simulink model "RSC_RRT"  (R2012b)
settings: Solver=ode3  StartTime=0.0  StopTime=10  FixedStep=.05  RelTol=1e-3
InitFcn:
  | a2g = 1/9.81;
  | r2d = 180/pi;
  | K_sr = 15.97;
  | neutral_steer = 104;
  | s2t = (pi/180)*(1/K_sr);
  | A_kt =[         0         0         0         0         0         0
  |          0   -3.5058   -1.6990  -25.6114   -2.2435         0
  |          0    2.2782   -4.2575  -64.1772   -5.6218         0
  |          0         0    1.0000         0         0         0
  |          0   -0.0158    0.0295    0.4442   -4.1900         0
  |          0         0         0         0    1.0000         0];
  | 
  | 
  | B_kt =[0
  |    23.7845
  |   -16.0342
  |          0
  |    17.5770
  |          0];
  | 
  | load MPC_test_2
undefined symbols (not defined in the file or in its folder): CR, DiscIntNeverNeededParam, serial
libraries: instrumentlib x3, mpclib x1, simulink x1, realtime_pacer_lib x1
settings Model: BufferReuse=off  Creator=TCA  LastModifiedBy=Thomas
settings DataIOCC: SignalLoggingSaveFormat=ModelDataLogs
settings OptimizationCC: BlockReduction=off  InlineParams=on  BufferReuse=off  InitFltsAndDblsToZero=on
settings DebuggingCC: ReadBeforeWriteMsg=DisableAll  AlgebraicLoopMsg=none  SolverPrmCheckMsg=none  FcnCallInpInsideContextMsg=UseLocalSettings  UnconnectedInputMsg=none  UnconnectedOutputMsg=none  UnconnectedLineMsg=none  StrictBusMsg=Warning
settings SFSimCC: SimParseCustomCode=off
settings RTWCC: TargetLang=C++
settings GRTTargetCC: CombineOutputUpdateFcns=off  GRTInterface=on

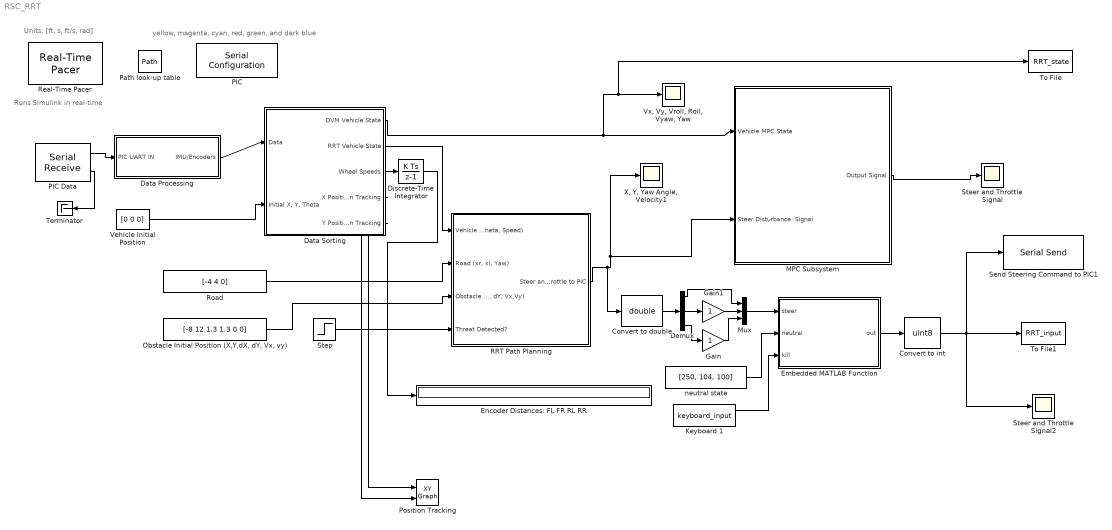
== system RSC_RRT ==
  note: Runs Simulink
      |  in real-time
  note: Units: [ft, s, ft/s, rad]
  note: yellow, magenta, cyan, red, green, and dark blue
  Convert to double : DataTypeConversion  OutDataTypeStr=double  SampleTime=0.05  SaturateOnIntegerOverflow=on  RndMeth=Zero
  Convert to int : DataTypeConversion  OutDataTypeStr=uint8  SampleTime=0.05  SaturateOnIntegerOverflow=on  RndMeth=Zero
  Data Processing : Subsystem
  Data Sorting : Subsystem
  Demux : Demux  Outputs=3
  Discrete-Time Integrator : DiscreteIntegrator  SampleTime=0.05  ICPrevOutput=DiscIntNeverNeededParam  ICPrevScaledInput=DiscIntNeverNeededParam
  Embedded MATLAB Function : MATLAB Function  TreatAsAtomicUnit=on
  Encoder Distances: FL FR RL RR : Display
  Gain : Gain
  Gain1 : Gain
  Keyboard 1 : M-S-Function  FunctionName=keyboard_input  mask(Keyboard Input){}
      mask help: Keyboard Input
      mask Display: fprintf('Keyboard');
  MPC Subsystem : Subsystem
  Mux : Mux  Inputs=3
  "Obstacle Initial Position (X,Y,dX, dY, Vx, vy)" : Constant  Value=[-8 12 1.3 1.3 0 0]
  PIC : instrumentlib/Serial Configuration  Priority=-200000  ComPortMenu=<Please select a port...>  ComPort=COM5  ObjConstructor=serial('COM5');  BaudRate=9600  DataBits=8  Parity=none  StopBits=1  FlowControl=none  Timeout=10  ByteOrder=LittleEndian
  PIC Data : instrumentlib/Serial Receive  ComPortMenu=<Please select a port...>  ComPort=COM5  ObjConstructor=serial('COM5');  Terminator=CR ('\r')  DataSize="[1  16]"  DataType=uint8  EnableBlockingMode=off  ActionDataUnavailable=Output last received value  CustomValue=0  SampleTime=.05
  Path look-up table : DataStoreMemory  DataStoreName=Path  ReadBeforeWriteMsg=warning  WriteAfterWriteMsg=warning  WriteAfterReadMsg=warning  InitialValue=zeros(50, 6)  VectorParams1D=off
  Position Tracking : simulink/Sinks/XY Graph  xmin=-10  xmax=10  ymin=-10  ymax=50  st=-1
  RRT Path Planning : Subsystem
  Real-Time Pacer : realtime_pacer_lib/Real-Time Pacer  simTimePerRealTime=1
  Road : Constant  Value=[-4 4 0]
  Send Steering Command to PIC1 : instrumentlib/Serial Send  ComPortMenu=<Please select a port...>  ComPort=COM5  ObjConstructor=serial('COM5');  Header=250  Terminator=<none>  EnableBlockingMode=off
  Steer and Throttle Signal : Scope
      settings: TimeRange=10  YMin=50  YMax=250  SaveName=ScopeData3
  Steer and Throttle Signal2 : Scope
      settings: TimeRange=10  YMin=50  YMax=250  SaveName=ScopeData4
  Step : Step  Time=2  SampleTime=0
  Terminator : Terminator
  To File : ToFile  Filename=RRT_state  MatrixName=RRT_state  SaveFormat=Timeseries
  To File1 : ToFile  Filename=RRT_input  MatrixName=RRT_input  SaveFormat=Timeseries
  Vehicle Initial Position : Constant  Value=[0 0 0]  VectorParams1D=off
  "Vx, Vy, Vroll, Roll, Vyaw, Yaw" : Scope
      settings: TimeRange=10  YMax=30  SaveName=ScopeData2
  "X, Y, Yaw Angle, Velocity1" : Scope
      settings: TimeRange=10  YMax=30  SaveName=ScopeData6
  neutral state : Constant  Value=[250, 104, 100]
  wires:
  PIC Data/2 -> Terminator/1
  Vehicle Initial Position/1 -> Data Sorting/2("Initial X, Y, Theta")
  PIC Data/1 -> Data Processing/1(PIC UART IN)
  Data Processing/1(IMU/Encoders) -> Data Sorting/1(Data)
  Discrete-Time Integrator/1 -> Encoder Distances: FL FR RL RR/1
  Data Sorting/3(Wheel Speeds) -> Discrete-Time Integrator/1
  Data Sorting/4(X Position Tracking) -> Position Tracking/1
  Data Sorting/5(Y Position Tracking) -> Position Tracking/2
  Data Sorting/1(DVM Vehicle State) -> MPC Subsystem/1(Vehicle MPC State), "Vx, Vy, Vroll, Roll, Vyaw, Yaw"/1, To File/1
  MPC Subsystem/1(Output Signal) -> Steer and Throttle Signal/1
  RRT Path Planning/1(Steer and Throttle to PIC) -> "X, Y, Yaw Angle, Velocity1"/1, MPC Subsystem/2(Steer Disturbance  Signal), Convert to double/1
  neutral state/1 -> Embedded MATLAB Function/2(neutral)
  Keyboard 1/1 -> Embedded MATLAB Function/3(kill)
  Embedded MATLAB Function/1(out) -> Convert to int/1
  Convert to int/1 -> Send Steering Command to PIC1/1, To File1/1, Steer and Throttle Signal2/1
  Convert to double/1 -> Demux/1
  Demux/3 -> Gain/1
  Gain/1 -> Mux/3
  Demux/1 -> Mux/1
  Mux/1 -> Embedded MATLAB Function/1(steer)
  Demux/2 -> Gain1/1
  Gain1/1 -> Mux/2
  Step/1 -> RRT Path Planning/4(Threat Detected?)
  "Obstacle Initial Position (X,Y,dX, dY, Vx, vy)"/1 -> RRT Path Planning/3("Obstacle Array (X,Y,dX, dY, Vx,Vy)")
  Road/1 -> RRT Path Planning/2("Road (xr, xl, Yaw)")
  Data Sorting/2(RRT Vehicle State) -> RRT Path Planning/1("Vehicle State (X,Y, Theta, Speed)")

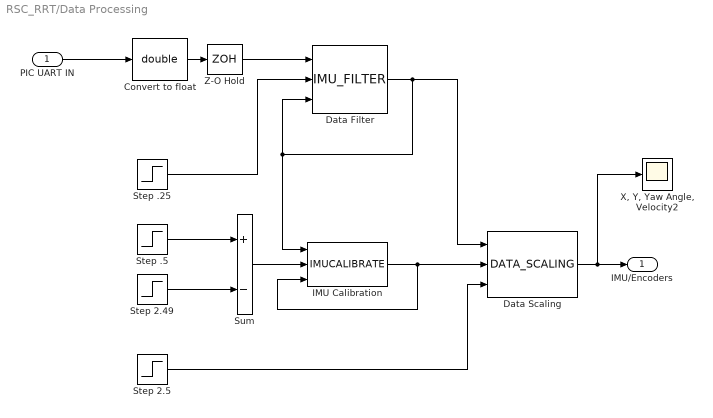
== system RSC_RRT/Data Processing ==
  PIC UART IN : Inport
  Convert to float : DataTypeConversion  OutDataTypeStr=double  SaturateOnIntegerOverflow=on  RndMeth=Zero
  Data Filter : M-S-Function  FunctionName=IMU_FILTER  Parameters=3
  "Data Scaling " : M-S-Function  FunctionName=DATA_SCALING  Parameters=3
  IMU Calibration : M-S-Function  FunctionName=IMUCALIBRATE  Parameters=3
  Step .25 : Step  Time=.25  SampleTime=0
  Step .5 : Step  Time=.5  SampleTime=0
  Step 2.49 : Step  Time=2.49  SampleTime=0
  Step 2.5 : Step  Time=2.5  SampleTime=0
  Sum : Sum  Inputs=+-
  "X, Y, Yaw Angle, Velocity2" : Scope
      settings: TimeRange=10  YMax=30  SaveName=ScopeData9
  Z-O Hold : ZeroOrderHold  SampleTime=0.05
  IMU/Encoders : Outport
  wires:
  Convert to float/1 -> Z-O Hold/1
  Data Filter/1 -> "Data Scaling "/1, IMU Calibration/1, Data Filter/3
  IMU Calibration/1 -> IMU Calibration/3, "Data Scaling "/2
  Step .5/1 -> Sum/1
  Step 2.49/1 -> Sum/2
  Z-O Hold/1 -> Data Filter/1
  Step .25/1 -> Data Filter/2
  Sum/1 -> IMU Calibration/2
  Step 2.5/1 -> "Data Scaling "/3
  "Data Scaling "/1 -> IMU/Encoders/1, "X, Y, Yaw Angle, Velocity2"/1
  PIC UART IN/1 -> Convert to float/1

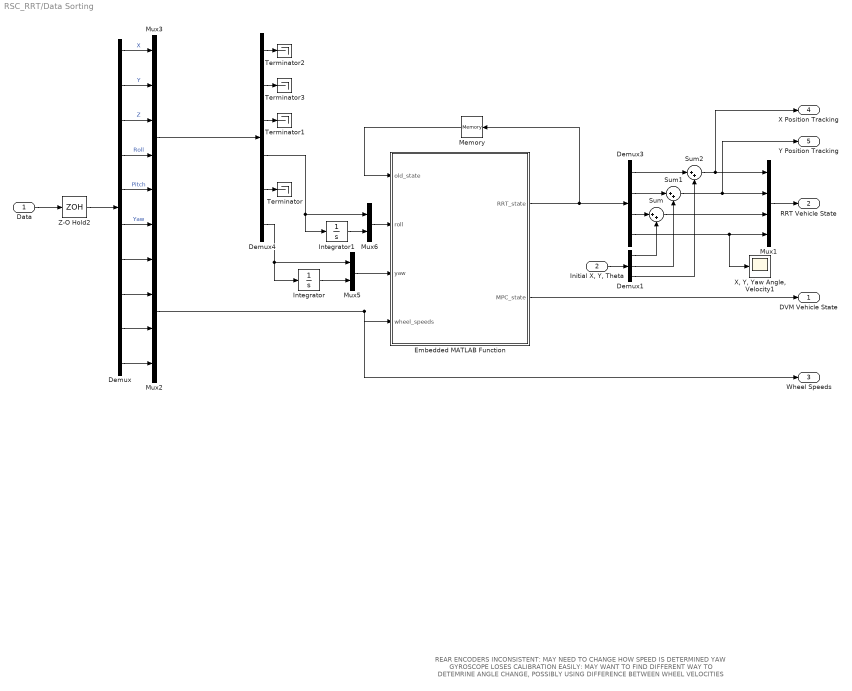
== system RSC_RRT/Data Sorting ==
  note: REAR ENCODERS INCONSISTENT: MAY NEED TO CHANGE HOW SPEED IS DETERMINED
      | YAW GYROSCOPE LOSES CALIBRATION EASILY: MAY WANT TO FIND DIFFERENT WAY TO DETEMRINE
      | ANGLE CHANGE, POSSIBLY USING DIFFERENCE BETWEEN WHEEL VELOCITIES
  Data : Inport
  "Initial X, Y, Theta" : Inport  Port=2
  Demux : Demux  Outputs=10
  Demux1 : Demux  Outputs=3
  Demux3 : Demux
  Demux4 : Demux  Outputs=6
  Embedded MATLAB Function : MATLAB Function  TreatAsAtomicUnit=on
  Integrator : Integrator
  Integrator1 : Integrator
  Memory : Memory  InheritSampleTime=on
  Mux1 : Mux
  Mux2 : Mux
  Mux3 : Mux  Inputs=6
  Mux5 : Mux  Inputs=2
  Mux6 : Mux  Inputs=2
  Sum : Sum  Inputs=|++
  Sum1 : Sum  Inputs=|++
  Sum2 : Sum  Inputs=|++
  Terminator{,1..3} (4 alike) : Terminator
  "X, Y, Yaw Angle, Velocity1" : Scope
      settings: TimeRange=10  YMax=30  SaveName=ScopeData7
  Z-O Hold2 : ZeroOrderHold  SampleTime=0.05
  DVM Vehicle State : Outport
  RRT Vehicle State : Outport  Port=2
  Wheel Speeds : Outport  Port=3
  X Position Tracking : Outport  Port=4
  Y Position Tracking : Outport  Port=5
  wires:
  Data/1 -> Z-O Hold2/1
  "Initial X, Y, Theta"/1 -> Demux1/1
  Memory/1 -> Embedded MATLAB Function/1(old_state)
  Embedded MATLAB Function/1(RRT_state) -> Memory/1, Demux3/1
  Demux/6 -> Mux3/6  "Yaw"
  Demux/1 -> Mux3/1  "X"
  Demux/2 -> Mux3/2  "Y"
  Mux3/1 -> Demux4/1
  Demux/3 -> Mux3/3  "Z"
  Demux/4 -> Mux3/4  "Roll"
  Demux/5 -> Mux3/5  "Pitch"
  Demux/7 -> Mux2/1
  Demux/8 -> Mux2/2
  Demux/9 -> Mux2/3
  Demux/10 -> Mux2/4
  Mux2/1 -> Embedded MATLAB Function/4(wheel_speeds), Wheel Speeds/1
  Z-O Hold2/1 -> Demux/1
  Demux1/1 -> Sum/2
  Demux1/2 -> Sum1/2
  Demux1/3 -> Sum2/2
  Demux3/2 -> Sum1/1
  Demux3/1 -> Sum2/1
  Demux3/3 -> Sum/1
  Sum2/1 -> Mux1/1, X Position Tracking/1
  Sum1/1 -> Mux1/2, Y Position Tracking/1
  Sum/1 -> Mux1/3
  Mux1/1 -> RRT Vehicle State/1
  Demux3/4 -> Mux1/4, "X, Y, Yaw Angle, Velocity1"/1
  Demux4/4 -> Integrator1/1, Mux6/1
  Demux4/6 -> Integrator/1, Mux5/1
  Integrator/1 -> Mux5/2
  Mux5/1 -> Embedded MATLAB Function/3(yaw)
  Integrator1/1 -> Mux6/2
  Mux6/1 -> Embedded MATLAB Function/2(roll)
  Demux4/5 -> Terminator/1
  Demux4/3 -> Terminator1/1
  Demux4/1 -> Terminator2/1
  Demux4/2 -> Terminator3/1
  Embedded MATLAB Function/2(MPC_state) -> DVM Vehicle State/1

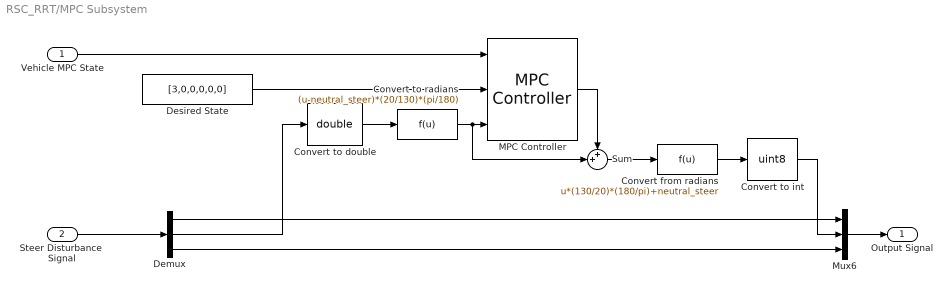
== system RSC_RRT/MPC Subsystem ==
  Vehicle MPC State : Inport
  Steer Disturbance  Signal : Inport  Port=2
  Convert from radians : Fcn  Expr=u*(130/20)*(180/pi)+neutral_steer
  Convert to double : DataTypeConversion  OutDataTypeStr=double  SampleTime=0.05  SaturateOnIntegerOverflow=on  RndMeth=Zero
  Convert to int : DataTypeConversion  OutDataTypeStr=uint8  SampleTime=0.05  SaturateOnIntegerOverflow=on  RndMeth=Zero
  Convert to radians : Fcn  Expr=(u-neutral_steer)*(20/130)*(pi/180)
  Demux : Demux  Outputs=3
  Desired State : Constant  Value=[3,0,0,0,0,0]
  MPC Controller : mpclib/MPC Controller  mpcobj=MPC_test_2  x0=[]  md_inport=on  mv_inport=off  lims_inport=off  switch_inport=off  ywt_inport=off  duwt_inport=off  rhoeps_inport=off  cost_outport=off  return_sequence=off  return_qpstatus=off  is_multiple=0  enable_value=0  n_mv=1  n_mo=6  n_md=1  n_ts=0.05  is_designfromscratch=0  ref_from_ws=off  ref_signal_name=[]  ref_preview=on  md_from_ws=off  md_signal_name=[]  md_preview=on  from_project=off  project_file=MPCtask.mat
  Mux6 : Mux  Inputs=3
  Sum : Sum  Inputs=++|
  Output Signal : Outport
  wires:
  Convert to double/1 -> Convert to radians/1
  Desired State/1 -> MPC Controller/2
  Convert to radians/1 -> MPC Controller/3, Sum/2
  MPC Controller/1 -> Sum/1
  Steer Disturbance  Signal/1 -> Demux/1
  Demux/2 -> Convert to double/1
  Demux/1 -> Mux6/1
  Convert from radians/1 -> Convert to int/1
  Demux/3 -> Mux6/3
  Mux6/1 -> Output Signal/1
  Vehicle MPC State/1 -> MPC Controller/1
  Sum/1 -> Convert from radians/1
  Convert to int/1 -> Mux6/2

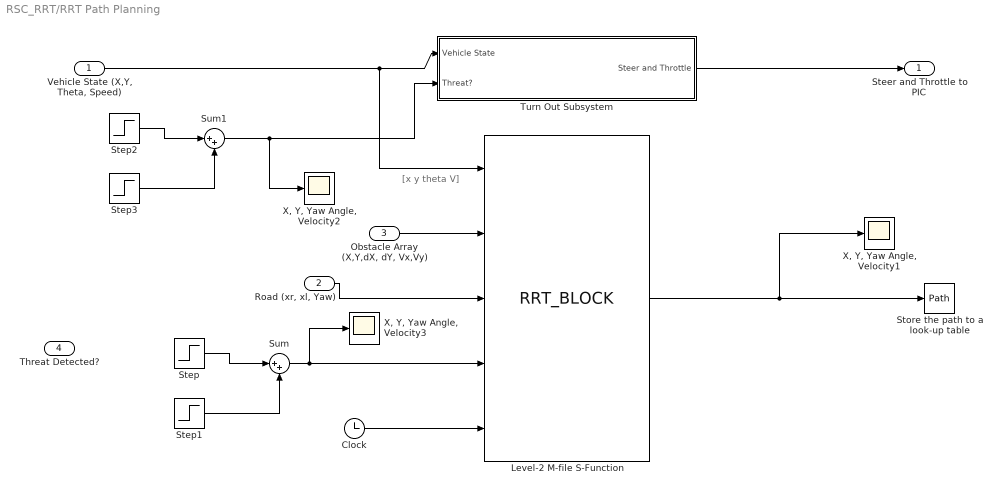
== system RSC_RRT/RRT Path Planning ==
  note: [x y theta V]
  "Vehicle State (X,Y, Theta, Speed)" : Inport
  "Road (xr, xl, Yaw)" : Inport  Port=2
  "Obstacle Array (X,Y,dX, dY, Vx,Vy)" : Inport  Port=3
  Threat Detected? : Inport  Port=4
  Clock : Clock
  Level-2 M-file S-Function : M-S-Function  FunctionName=RRT_BLOCK  Parameters=6
  Step : Step  Time=2.1  After=0  SampleTime=0
  Step1 : Step  Time=2.2  After=0  SampleTime=0
  Step2 : Step  Time=3  SampleTime=0
  Step3 : Step  Time=7  After=-1  SampleTime=0
  Store the path to a look-up table : DataStoreWrite  DataStoreName=Path
  Sum : Sum  Inputs=|++
  Sum1 : Sum  Inputs=|++
  Turn Out Subsystem : Subsystem
  "X, Y, Yaw Angle, Velocity1" : Scope
      settings: TimeRange=10  YMax=30
  "X, Y, Yaw Angle, Velocity2" : Scope
      settings: TimeRange=10  YMax=30
  "X, Y, Yaw Angle, Velocity3" : Scope
      settings: TimeRange=10  YMax=30  SaveName=ScopeData5
  Steer and Throttle to PIC : Outport
  wires:
  Step/1 -> Sum/1
  Level-2 M-file S-Function/1 -> Store the path to a look-up table/1, "X, Y, Yaw Angle, Velocity1"/1
  Clock/1 -> Level-2 M-file S-Function/5
  "Vehicle State (X,Y, Theta, Speed)"/1 -> Level-2 M-file S-Function/1, Turn Out Subsystem/1(Vehicle State)
  "Obstacle Array (X,Y,dX, dY, Vx,Vy)"/1 -> Level-2 M-file S-Function/2
  Turn Out Subsystem/1(Steer and Throttle) -> Steer and Throttle to PIC/1
  "Road (xr, xl, Yaw)"/1 -> Level-2 M-file S-Function/3
  Sum/1 -> Level-2 M-file S-Function/4, "X, Y, Yaw Angle, Velocity3"/1
  Step2/1 -> Sum1/1
  Step3/1 -> Sum1/2
  Sum1/1 -> Turn Out Subsystem/2(Threat?), "X, Y, Yaw Angle, Velocity2"/1
  Step1/1 -> Sum/2

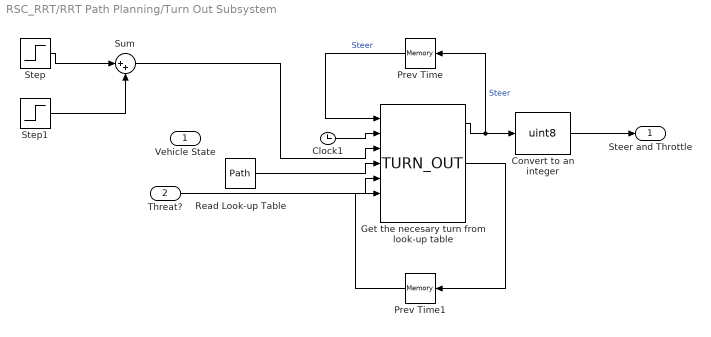
== system RSC_RRT/RRT Path Planning/Turn Out Subsystem ==
  Vehicle State : Inport
  Threat? : Inport  Port=2
  Clock1 : Clock
  Convert to an integer : DataTypeConversion  OutDataTypeStr=uint8  SampleTime=.05  SaturateOnIntegerOverflow=on  RndMeth=Zero
  Get the necesary turn from look-up table : M-S-Function  FunctionName=TURN_OUT  Parameters=4
  Prev Time : Memory  X0=[250 104 100]
  Prev Time1 : Memory
  Read Look-up Table : DataStoreRead  DataStoreName=Path  SampleTime=0
  Step : Step  Time=0  After=17  SampleTime=0
  Step1 : Step  Time=5  After=-2  SampleTime=0
  Sum : Sum  Inputs=|++
  Steer and Throttle : Outport
  wires:
  Get the necesary turn from look-up table/1 -> Convert to an integer/1, Prev Time/1  "Steer"
  Convert to an integer/1 -> Steer and Throttle/1
  Prev Time/1 -> Get the necesary turn from look-up table/1  "Steer"
  Get the necesary turn from look-up table/2 -> Prev Time1/1
  Clock1/1 -> Get the necesary turn from look-up table/2
  Read Look-up Table/1 -> Get the necesary turn from look-up table/4
  Prev Time1/1 -> Get the necesary turn from look-up table/6
  Threat?/1 -> Get the necesary turn from look-up table/5
  Step/1 -> Sum/1
  Step1/1 -> Sum/2
  Sum/1 -> Get the necesary turn from look-up table/3

== matlab function RSC_RRT/Data Sorting/Embedded MATLAB Function ==
  data: old_state input; roll input; yaw input; wheel_speeds input; RRT_state output; MPC_state output
% function [x,y,theta,velocity, TESTING] = fcn(x_old,y_old,theta_old,yaw_rate_IMU,Vl_old,Vr_old)
% %#eml
% 
% deltaK = 0.05;
% 
% delta_theta_enc = (Vr_old - Vl_old)*(12/10)*deltaK;
% delta_theta_imu = yaw_rate_IMU*deltaK;
% delta_theta = (delta_theta_enc+delta_theta_imu)/2;
% 
% theta = theta_old + delta_theta;
% 
% velocity = (Vl_old + Vr_old)/2;
% 
% x = x_old + velocity*-1*sin(theta_old)*deltaK;
% y = y_old + velocity*cos(theta_old)*deltaK;

%NEW AWESOME DATA SORTING
function [RRT_state,MPC_state]  = data_sorting(old_state,roll,yaw, wheel_speeds)
%#eml
deltaK = 0.05;

x_old = old_state(1);
y_old = old_state(2);

velocity = (wheel_speeds(1) + wheel_speeds(2) + wheel_speeds(3) + wheel_speeds(4))/4;

Phi_d = roll(1);
Phi = roll(2);
Psi_d = yaw(1);
Psi = yaw(2);
Vx = velocity*sin(Psi);
Vy = velocity*cos(Psi); 

x = x_old - Vx*deltaK;
y = y_old + Vy*deltaK;

MPC_state = [Vx*(1/3.28), Vy*(1/3.28), Phi_d, Phi, Psi_d, Psi]';
RRT_state = [x, y, Psi, velocity]';

== matlab function RSC_RRT/Embedded MATLAB Function ==
  data: steer input; out output; neutral input; kill input
function out = fcn(steer,neutral,kill)
%#eml

if(kill)
    out = neutral;
else
    out = steer;
end

%end
